simulink model "Ex6_5"  (Simulink 6.0)
settings: Solver=FixedStepDiscrete  SolverMode=SingleTasking  StartTime=0.0  StopTime=Ts*10  FixedStep=Ts  RelTol=1e-3  AbsTol=1e-6
values from neighbouring files (symbols this model uses):
  Ampl = 10^(Amp_dB/20)-pi/1024    (= 0.313159804441)    [Ex6_2Launch.m]
  finrad = Fin*2*pi    (= 11888.3511061)    [Ex6_2Launch.m]
  gainerr1 = A0/(A0+1+C1/C2)    (= 0.9999800004)    [Ex6_2Launch.m]
  gainerr2 = A0/(A0+1+C1/C2)    (= 0.9999800004)    [Ex6_2Launch.m]
  phaseerr1 = (1+A0)*C2/((1+A0)*C2+C1)    (= 0.9999900002)    [Ex6_2Launch.m]
  Ts = 1/Fs    (= 5e-07)    [Ex6_2Launch.m]
settings Model: Creator=francomaloberti  LastModifiedBy=Cri  ExtModeAutoUpdateStatusClock=off
settings DataIOCC: LimitDataPoints=off  SignalLoggingName=sigsOut
settings OptimizationCC: BooleanDataType=off  InlineInvariantSignals=off
settings DebuggingCC: SolverPrmCheckMsg=none
settings HardwareCC: TargetUnknown=on

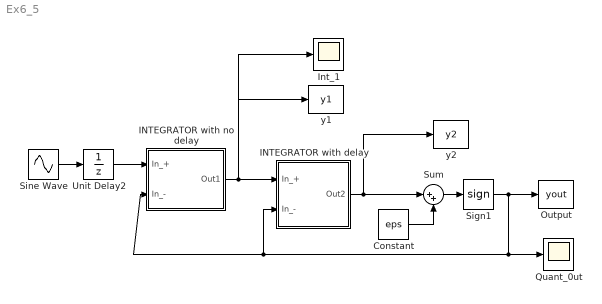
== system Ex6_5 ==
  Constant : Constant  Value=eps
  INTEGRATOR with delay : Subsystem
      mask Display:
      | patch([10 40 10 10], [0 20 40 0],[1 0 1])
      | plot([10 40 10 10], [0 20 40 0])
      | plot([0 10], [8 8])
      | plot([0 10], [28 28])
      | dpoly([0 1], [1 -1], 'z-')
      | port_label('input', 1, '+')
      | port_label('input', 2, '-')
  INTEGRATOR with no delay : Subsystem
      mask Display:
      | patch([10 40 10 10], [0 20 40 0],[0 1 1])
      | plot([10 40 10 10], [0 20 40 0])
      | plot([0 10], [8 8])
      | plot([0 10], [28 28])
      | dpoly([1], [1 -1], 'z-')
      | port_label('input', 1, '+')
      | port_label('input', 2, '-')
  Int_1 : Scope
      settings: TimeRange=0.003  YMin=-0.4  YMax=0.4  SaveName=ScopeData3
  Output : ToWorkspace  VariableName=yout  SampleTime=-1  SaveFormat=Array
  Quant_0ut : Scope
  Sign1 : Signum
  Sine Wave : Sin  Amplitude=Ampl  Frequency=finrad  SampleTime=0
  Sum : Sum  Inputs=|++
  Unit Delay2 : UnitDelay  SampleTime=Ts
  y1 : ToWorkspace  VariableName=y1  SampleTime=-1  SaveFormat=Array
  y2 : ToWorkspace  VariableName=y2  SampleTime=-1  SaveFormat=Array
  wires:
  Unit Delay2/1 -> INTEGRATOR with no delay/1(In_+)
  INTEGRATOR with delay/1(Out2) -> y2/1, Sum/1
  INTEGRATOR with no delay/1(Out1) -> Int_1/1, y1/1, INTEGRATOR with delay/1(In_+)
  Sum/1 -> Sign1/1
  Sign1/1 -> Quant_0ut/1, INTEGRATOR with delay/2(In_-), INTEGRATOR with no delay/2(In_-), Output/1
  Constant/1 -> Sum/2
  Sine Wave/1 -> Unit Delay2/1

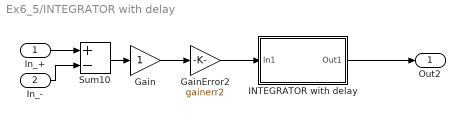
== system Ex6_5/INTEGRATOR with delay ==
  In_+ : Inport  Port=1  LatchInput=off
  In_- : Inport  Port=2  LatchInput=off
  Gain : Gain  SaturateOnIntegerOverflow=on
  GainError2 : Gain  Gain=gainerr2  SaturateOnIntegerOverflow=on
  INTEGRATOR with delay : Subsystem
      mask Display:
      | patch([0 20 0 0], [0 10 20 0],[0 1 0])
      | text(5,10,'\bf\int','texmode','on')
      | plot([0 20 0 0], [0 10 20 0])
  Sum10 : Sum  Inputs=+-  SaturateOnIntegerOverflow=on  InputSameDT=on
  Out2 : Outport
  wires:
  Gain/1 -> GainError2/1
  Sum10/1 -> Gain/1
  In_-/1 -> Sum10/2
  In_+/1 -> Sum10/1
  GainError2/1 -> INTEGRATOR with delay/1(In1)
  INTEGRATOR with delay/1(Out1) -> Out2/1

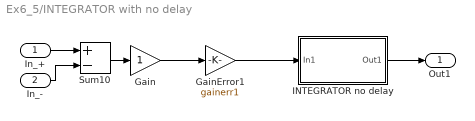
== system Ex6_5/INTEGRATOR with no delay ==
  In_+ : Inport  Port=1  LatchInput=off
  In_- : Inport  Port=2  LatchInput=off
  Gain : Gain  SaturateOnIntegerOverflow=on
  GainError1 : Gain  Gain=gainerr1  SaturateOnIntegerOverflow=on
  INTEGRATOR no delay : Subsystem
      mask Display:
      | patch([0 20 0 0], [0 10 20 0],[0 1 1])
      | text(5,10,'\bf\int','texmode','on')
      | plot([0 20 0 0], [0 10 20 0])
  Sum10 : Sum  Inputs=+-  SaturateOnIntegerOverflow=on  InputSameDT=on
  Out1 : Outport
  wires:
  Gain/1 -> GainError1/1
  Sum10/1 -> Gain/1
  In_-/1 -> Sum10/2
  In_+/1 -> Sum10/1
  GainError1/1 -> INTEGRATOR no delay/1(In1)
  INTEGRATOR no delay/1(Out1) -> Out1/1

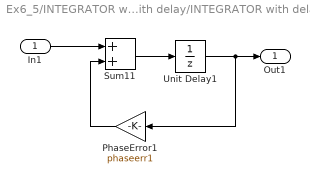
== system Ex6_5/INTEGRATOR with delay/INTEGRATOR with delay ==
  In1 : Inport  Port=1  LatchInput=off
  PhaseError1 : Gain  Orientation=left  Gain=phaseerr1  SaturateOnIntegerOverflow=on
  Sum11 : Sum  SaturateOnIntegerOverflow=on  InputSameDT=on
  Unit Delay1 : UnitDelay  SampleTime=Ts
  Out1 : Outport
  wires:
  In1/1 -> Sum11/1
  Sum11/1 -> Unit Delay1/1
  PhaseError1/1 -> Sum11/2
  Unit Delay1/1 -> Out1/1, PhaseError1/1

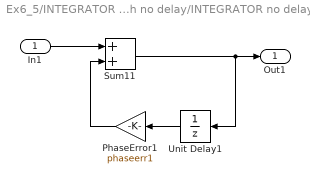
== system Ex6_5/INTEGRATOR with no delay/INTEGRATOR no delay ==
  In1 : Inport  Port=1  LatchInput=off
  PhaseError1 : Gain  Orientation=left  Gain=phaseerr1  SaturateOnIntegerOverflow=on
  Sum11 : Sum  SaturateOnIntegerOverflow=on  InputSameDT=on
  Unit Delay1 : UnitDelay  Orientation=left  SampleTime=Ts
  Out1 : Outport
  wires:
  PhaseError1/1 -> Sum11/2
  Sum11/1 -> Unit Delay1/1, Out1/1
  Unit Delay1/1 -> PhaseError1/1
  In1/1 -> Sum11/1
